simulink model "TankModel_sim"  (R2020b)
settings: Solver=VariableStepAuto  StartTime=0.0  StopTime=Endtime  RelTol=1e-3
values from neighbouring files (symbols this model uses):
  C = D^2/4*pi    (= 0.196349540849)    [Tanksim.m]
  q1 = 1e-3    (= 0.001)    [Tanksim.m]
  R = 500    [Tanksim.m]
settings Model: Creator=yuto  LastModifiedBy=yuto

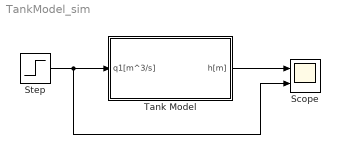
== system TankModel_sim ==
  Scope : Scope  NumInputPorts=2
  Step : Step  After=q1  SampleTime=0
  Tank Model : Subsystem
  wires:
  Step/1 -> Scope/2, Tank Model/1(q1[m^3/s])
  Tank Model/1(h[m]) -> Scope/1

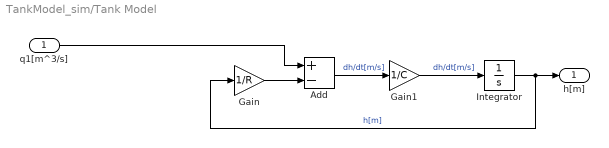
== system TankModel_sim/Tank Model ==
  q1[m^3/s] : Inport
  Add : Sum  Inputs=+-
  Gain : Gain  Gain=1/R
  Gain1 : Gain  Gain=1/C
  Integrator : Integrator
  h[m] : Outport
  wires:
  Integrator/1 -> Gain/1, h[m]/1  "h[m]"
  Add/1 -> Gain1/1  "dh/dt[m/s]"
  Gain/1 -> Add/2
  q1[m^3/s]/1 -> Add/1
  Gain1/1 -> Integrator/1  "dh/dt[m/s]"
